simulink model "flyback_simulation_V2"  (R2022b)
settings: Solver=VariableStepAuto  StartTime=0.0  StopTime=0.01  RelTol=1e-3
libraries: spsSeriesRLCBranchLib x2, spsCurrentMeasurementLib x1, spsDCVoltageSourceLib x1, spsDiodeLib x1, spsMosfetLib x1, spsMultiWindingTransformerLib x1, spsVoltageMeasurementLib x1, spspowerguiLib x1
settings Model: Creator=basak  LastModifiedBy=basak

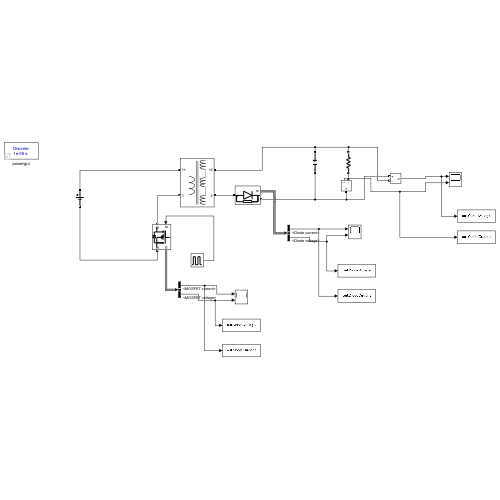
[thumbnail: Simulink's stored preview of the top-level diagram]
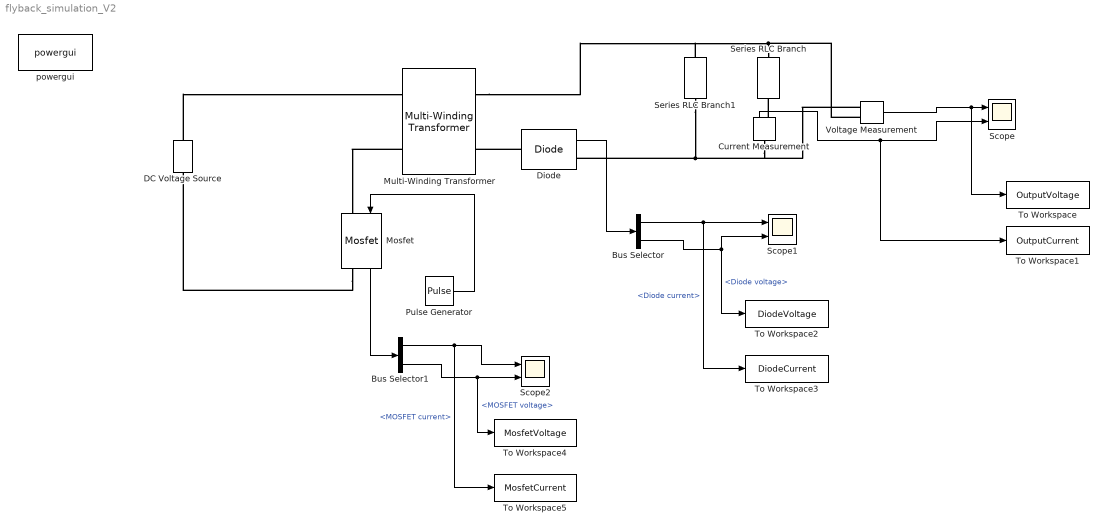
== system flyback_simulation_V2 ==
  Bus Selector : BusSelector  OutputSignals=Diode current,Diode voltage
  Bus Selector1 : BusSelector  OutputSignals=MOSFET current,MOSFET voltage
  Current Measurement : spsCurrentMeasurementLib/Current Measurement  PhasorSimulation=off  OutputType=Complex  PSBequivalent=0
  DC Voltage Source : spsDCVoltageSourceLib/DC Voltage Source  Amplitude=15  Measurements=None
  Diode : spsDiodeLib/Diode  Ron=1e-9  Lon=0  Vf=0  IC=0  UseSnubber=0  Rs=500  Cs=250e-9  Measurements=on
  Mosfet : spsMosfetLib/Mosfet  Ron=1e-9  Lon=0  Rd=1e-9  Vfd=0  IC=0  Rs=1e5  Cs=inf  Measurements=on
  Multi-Winding Transformer : spsMultiWindingTransformerLib/Multi-Winding Transformer  LeftWindings=1  RightWindings=1  TappedWindings=no taps  NumberOfTaps=2  SetSaturation=off  Hysteresis=off  DataFile='hysteresis.mat'  Measurements=None  UNITS=SI  NominalPower=[48 1e5]  NominalVoltages=[48 48]  WindingResistances=[0 0]  WindingInductances=[0 0]  Rm=Inf  Lm=3.375e-6  Saturation=[0 0;0.50001 0.00072952;208.33 0.00092405]  SpecifyInitialFlux=off  InitialFlux=0  BreakLoop=off  DiscreteSolver=Trapezoidal iterative  DataType=on  TransfoNumber=1
  Pulse Generator : DiscretePulseGenerator  PulseType=Time based  Period=1e-5  PulseWidth=40
  Scope : Scope  NumInputPorts=2
  Scope1 : Scope  NumInputPorts=2
  Scope2 : Scope  NumInputPorts=2
  Series RLC Branch : spsSeriesRLCBranchLib/Series RLC Branch  LConnTagsString=__new0  RConnTagsString=__new0  BranchType=R  Resistance=48  Inductance=1e-3  SetiL0=off  InitialCurrent=0  Capacitance=1e-6  Setx0=off  InitialVoltage=0  Measurements=None
  Series RLC Branch1 : spsSeriesRLCBranchLib/Series RLC Branch  LConnTagsString=__new0  RConnTagsString=__new0  BranchType=C  Resistance=1  Inductance=1e-3  SetiL0=off  InitialCurrent=0  Capacitance=4.7e-6  Setx0=off  InitialVoltage=0  Measurements=None
  To Workspace : ToWorkspace  VariableName=OutputVoltage  SaveFormat=Timeseries  SampleTime=-1
  To Workspace1 : ToWorkspace  VariableName=OutputCurrent  SaveFormat=Timeseries  SampleTime=-1
  To Workspace2 : ToWorkspace  VariableName=DiodeVoltage  SaveFormat=Timeseries  SampleTime=-1
  To Workspace3 : ToWorkspace  VariableName=DiodeCurrent  SaveFormat=Timeseries  SampleTime=-1
  To Workspace4 : ToWorkspace  VariableName=MosfetVoltage  SaveFormat=Timeseries  SampleTime=-1
  To Workspace5 : ToWorkspace  VariableName=MosfetCurrent  SaveFormat=Timeseries  SampleTime=-1
  Voltage Measurement : spsVoltageMeasurementLib/Voltage Measurement  PhasorSimulation=off  OutputType=Complex  PSBequivalent=0
  powergui : spspowerguiLib/powergui  Priority=1  SimulationMode=Discrete  SampleTime=1e-8  frequency=60  Iterations=50  frequencyindice=0  Pbase=100e6  ErrMax=1e-4  UnitsV=kV  UnitsW=MW  buscounter=0  FunctionMessages=off  echomessages=off  EnableUseOfTLC=off  CurrentSourceSwitches=off  DisableSnubberDevices=off  DisableRonSwitches=off  DisableVfSwitches=off  DisplayEquations=off  AutomaticDiscreteSolvers=off  SolverType=Tustin/Backward Euler (TBE)  Interpol=off  ExternalGateDelay=off  methode=off  Ts=100  x0status=blocks  SPID=on  SwTol=0  HookPort=off  NonlinearTolerance=1e-4  nMaxIteration=100  ContinueOnMaxIteration=off  RestoreLinks=warning  ResistiveCurrentMeasurement=off  Frange=[0:2:500]  Ylog=off  Xlog=on  ShowGrid=off  save=off  variable=ZData  structure=0  ZoomFFT=off  StartTime=0.0  cycles=1  DisplayStyle=1  fundamental=60  FreqAxis=off  MaxFrequency=1000  frequencyindicesteady=1  RmsSteady=1  display=off
  wires:
  Bus Selector/2 -> To Workspace2/1, Scope1/2  "<Diode voltage>"
  Bus Selector1/2 -> To Workspace4/1, Scope2/2  "<MOSFET voltage>"
  Bus Selector/1 -> To Workspace3/1, Scope1/1  "<Diode current>"
  Bus Selector1/1 -> To Workspace5/1, Scope2/1  "<MOSFET current>"
  Mosfet/1 -> Bus Selector1/1
  Voltage Measurement/1 -> To Workspace/1, Scope/1
  Current Measurement/1 -> To Workspace1/1, Scope/2
  Diode/1 -> Bus Selector/1
  Pulse Generator/1 -> Mosfet/1
  connections:
  Series RLC Branch1/LConn1 -- Diode/RConn1 -- Current Measurement/LConn1 -- Voltage Measurement/LConn1
  Series RLC Branch/RConn1 -- Series RLC Branch1/RConn1 -- Multi-Winding Transformer/RConn1 -- Voltage Measurement/LConn2
  Diode/LConn1 -- Multi-Winding Transformer/RConn2
  DC Voltage Source/RConn1 -- Multi-Winding Transformer/LConn1
  Multi-Winding Transformer/LConn2 -- Mosfet/LConn1
  Current Measurement/RConn1 -- Series RLC Branch/LConn1
  Mosfet/RConn1 -- DC Voltage Source/LConn1
